simulink model "diapo_model"  (R2014a)
settings: Solver=ode45  StartTime=0.0  StopTime=0.03  RelTol=1e-3
values from neighbouring files (symbols this model uses):
  C = 4.6e-5    (= 4.6e-05)    [tipe_vars.m]
  K = (pi*Rproj^4*gam*(mu*n)^2)/(8*m*Rbob^2)    (= 2.96114824556e-08)    [tipe_vars.m]
  L0 = 0.0015    [tipe_vars.m]
  Lbob = 0.06    [tipe_vars.m]
  Lproj = 0.025    [tipe_vars.m]
  R = 15    [tipe_vars.m]
  Rbob = 0.015    [tipe_vars.m]
  U0 = 800    [tipe_vars.m]
settings Model: Creator=jackhalford  LastModifiedBy=jackhalford
settings SolverCC: ShapePreserveControl=EnableAll  ZeroCrossControl=DisableAll

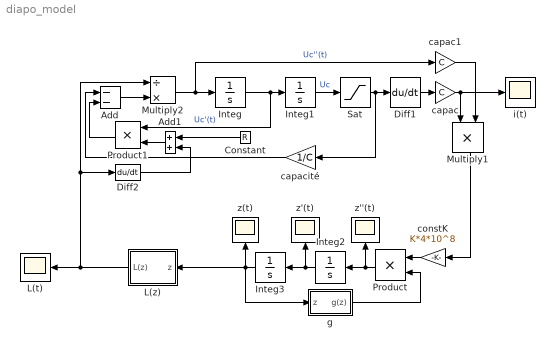
== system diapo_model ==
  Add : Sum  Inputs=--
  Add1 : Sum
  Constant : Constant  Value=R
  Diff1 : Derivative
  Diff2 : Derivative
  Integ : Integrator
  "Integ1 " : Integrator  InitialCondition=-U0
  Integ2 : Integrator  InitialCondition=8
  Integ3 : Integrator  InitialCondition=-(Lbob+Lproj)/2
  L(t) : Scope
      settings: TimeRange=0.003  YMin=-0.0425  YMax=-0.04235
  L(z) : Subsystem
  Multiply1 : Product  Inputs=**
  Multiply2 : Product  Inputs=/*
  Product : Product
  Product1 : Product
  Sat : Saturate  UpperLimit=10000  LowerLimit=-10000
  capac : Gain  Gain=C
  capac1 : Gain  Gain=C
  capacité : Gain  Gain=1/C
  constK : Gain  Gain=K*4*10^8
  g : Subsystem
  i(t) : Scope
      settings: TimeRange=0.005  YMin=0  YMax=80  SaveName=ScopeData17
  z''(t) : Scope
      settings: YMin=1.03225e-09  YMax=1.03675e-09  SaveName=ScopeData3
  z'(t) : Scope
      settings: TimeRange=0.03  YMin=720000  YMax=738000  SaveName=ScopeData13
  z(t) : Scope
      settings: TimeRange=0.003  YMin=-0.0425  YMax=-0.04235  SaveName=ScopeData4
  wires:
  capac/1 -> i(t)/1, Multiply1/1
  Multiply2/1 -> capac1/1, Integ/1  "Uc''(t)"
  Integ/1 -> Product1/1, "Integ1 "/1  "Uc'(t)"
  Product1/1 -> Add/2
  Add/1 -> Multiply2/2
  capacité/1 -> Add/1
  Diff1/1 -> capac/1
  "Integ1 "/1 -> Sat/1  "Uc"
  Sat/1 -> Diff1/1, capacité/1
  Product/1 -> Integ2/1, z''(t)/1
  Integ2/1 -> Integ3/1, z'(t)/1
  Integ3/1 -> z(t)/1, L(z)/1("z "), g/1("z ")
  capac1/1 -> Multiply1/2
  Multiply1/1 -> constK/1
  constK/1 -> Product/1
  g/1(g(z)) -> Product/2
  L(z)/1(L(z)) -> Multiply2/1, Diff2/1, L(t)/1
  Add1/1 -> Product1/2
  Constant/1 -> Add1/1
  Diff2/1 -> Add1/2

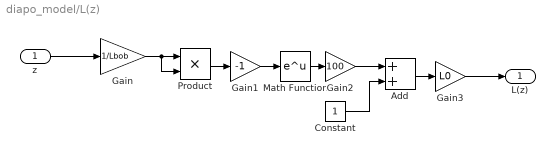
== system diapo_model/L(z) ==
  "z " : Inport
  Add : Sum
  Constant : Constant
  Gain : Gain  Gain=1/Lbob
  Gain1 : Gain  Gain=-1
  Gain2 : Gain  Gain=100
  Gain3 : Gain  Gain=L0
  Math Function : Math  SaturateOnIntegerOverflow=on
  Product : Product
  L(z) : Outport
  wires:
  "z "/1 -> Gain/1
  Gain/1 -> Product/2, Product/1
  Product/1 -> Gain1/1
  Gain1/1 -> Math Function/1
  Math Function/1 -> Gain2/1
  Gain2/1 -> Add/1
  Constant/1 -> Add/2
  Add/1 -> Gain3/1
  Gain3/1 -> L(z)/1

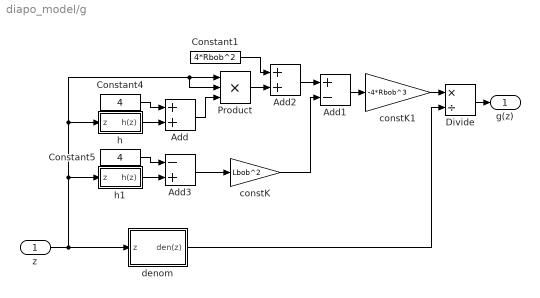
== system diapo_model/g ==
  "z " : Inport
  Add : Sum
  Add1 : Sum  Inputs=+-
  Add2 : Sum
  Add3 : Sum  Inputs=-+
  Constant1 : Constant  Value=4*Rbob^2
  Constant4 : Constant  Value=4
  Constant5 : Constant  Value=4
  Divide : Product  Inputs=*/
  Product : Product  Inputs=3
  constK : Gain  Gain=Lbob^2
  constK1 : Gain  Gain=-4*Rbob^3
  denom : Subsystem
  "h " : Subsystem
  "h1 " : Subsystem
  g(z) : Outport
  wires:
  Add/1 -> Product/3
  "h "/1(h(z)) -> Add/2
  Add2/1 -> Add1/1
  Divide/1 -> g(z)/1
  "z "/1 -> denom/1("z "), "h "/1("z "), Product/2, Product/1, "h1 "/1("z ")
  Constant4/1 -> Add/1
  Product/1 -> Add2/2
  Constant1/1 -> Add2/1
  constK/1 -> Add1/2
  denom/1(den(z)) -> Divide/2
  Constant5/1 -> Add3/1
  "h1 "/1(h(z)) -> Add3/2
  Add3/1 -> constK/1
  constK1/1 -> Divide/1
  Add1/1 -> constK1/1

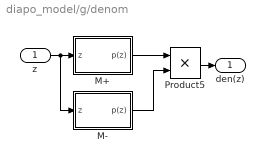
== system diapo_model/g/denom ==
  "z " : Inport
  M+ : Subsystem
  M- : Subsystem
  Product5 : Product
  den(z) : Outport
  wires:
  "z "/1 -> M-/1("z "), M+/1("z ")
  M+/1(p(z)) -> Product5/1
  M-/1(p(z)) -> Product5/2
  Product5/1 -> den(z)/1

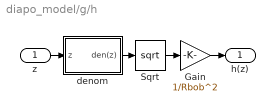
== system diapo_model/g/h  ==
  "z " : Inport
  Gain : Gain  Gain=1/Rbob^2
  Sqrt : Sqrt  SaturateOnIntegerOverflow=on
  denom : Subsystem
  h(z) : Outport
  wires:
  "z "/1 -> denom/1("z ")
  denom/1(den(z)) -> Sqrt/1
  Sqrt/1 -> Gain/1
  Gain/1 -> h(z)/1

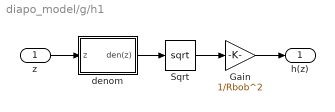
== system diapo_model/g/h1  ==
  "z " : Inport
  Gain : Gain  Gain=1/Rbob^2
  Sqrt : Sqrt  SaturateOnIntegerOverflow=on
  denom : Subsystem
  h(z) : Outport
  wires:
  "z "/1 -> denom/1("z ")
  denom/1(den(z)) -> Sqrt/1
  Sqrt/1 -> Gain/1
  Gain/1 -> h(z)/1

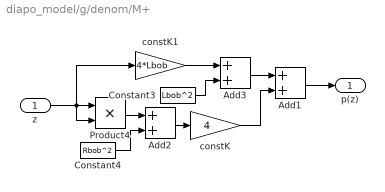
== system diapo_model/g/denom/M+ ==
  "z " : Inport
  Add1 : Sum
  Add2 : Sum
  Add3 : Sum
  Constant3 : Constant  Value=Lbob^2
  Constant4 : Constant  Value=Rbob^2
  Product4 : Product
  constK : Gain  Gain=4
  constK1 : Gain  Gain=4*Lbob
  p(z) : Outport
  wires:
  Product4/1 -> Add2/1
  Constant4/1 -> Add2/2
  Add2/1 -> constK/1
  constK1/1 -> Add3/1
  Constant3/1 -> Add3/2
  "z "/1 -> constK1/1, Product4/2, Product4/1
  Add3/1 -> Add1/1
  constK/1 -> Add1/2
  Add1/1 -> p(z)/1

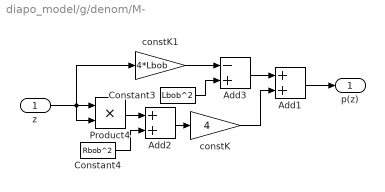
== system diapo_model/g/denom/M- ==
  "z " : Inport
  Add1 : Sum
  Add2 : Sum
  Add3 : Sum  Inputs=-+
  Constant3 : Constant  Value=Lbob^2
  Constant4 : Constant  Value=Rbob^2
  Product4 : Product
  constK : Gain  Gain=4
  constK1 : Gain  Gain=4*Lbob
  p(z) : Outport
  wires:
  Product4/1 -> Add2/1
  Constant4/1 -> Add2/2
  Add2/1 -> constK/1
  constK1/1 -> Add3/1
  Constant3/1 -> Add3/2
  "z "/1 -> constK1/1, Product4/2, Product4/1
  Add3/1 -> Add1/1
  constK/1 -> Add1/2
  Add1/1 -> p(z)/1

== system diapo_model/g/h /denom ==
  "z " : Inport
  M+ : Subsystem
  M- : Subsystem
  Product5 : Product
  den(z) : Outport
  wires:
  "z "/1 -> M-/1("z "), M+/1("z ")
  M+/1(p(z)) -> Product5/1
  M-/1(p(z)) -> Product5/2
  Product5/1 -> den(z)/1

== system diapo_model/g/h1 /denom ==
  "z " : Inport
  M+ : Subsystem
  M- : Subsystem
  Product5 : Product
  den(z) : Outport
  wires:
  "z "/1 -> M-/1("z "), M+/1("z ")
  M+/1(p(z)) -> Product5/1
  M-/1(p(z)) -> Product5/2
  Product5/1 -> den(z)/1

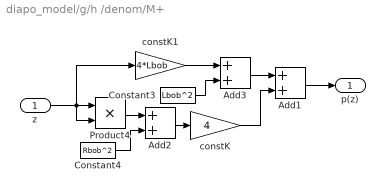
== system diapo_model/g/h /denom/M+ ==
  "z " : Inport
  Add1 : Sum
  Add2 : Sum
  Add3 : Sum
  Constant3 : Constant  Value=Lbob^2
  Constant4 : Constant  Value=Rbob^2
  Product4 : Product
  constK : Gain  Gain=4
  constK1 : Gain  Gain=4*Lbob
  p(z) : Outport
  wires:
  Product4/1 -> Add2/1
  Constant4/1 -> Add2/2
  Add2/1 -> constK/1
  constK1/1 -> Add3/1
  Constant3/1 -> Add3/2
  "z "/1 -> constK1/1, Product4/2, Product4/1
  Add3/1 -> Add1/1
  constK/1 -> Add1/2
  Add1/1 -> p(z)/1

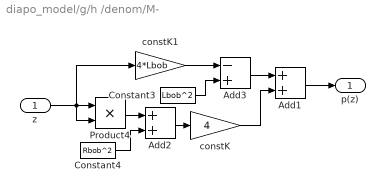
== system diapo_model/g/h /denom/M- ==
  "z " : Inport
  Add1 : Sum
  Add2 : Sum
  Add3 : Sum  Inputs=-+
  Constant3 : Constant  Value=Lbob^2
  Constant4 : Constant  Value=Rbob^2
  Product4 : Product
  constK : Gain  Gain=4
  constK1 : Gain  Gain=4*Lbob
  p(z) : Outport
  wires:
  Product4/1 -> Add2/1
  Constant4/1 -> Add2/2
  Add2/1 -> constK/1
  constK1/1 -> Add3/1
  Constant3/1 -> Add3/2
  "z "/1 -> constK1/1, Product4/2, Product4/1
  Add3/1 -> Add1/1
  constK/1 -> Add1/2
  Add1/1 -> p(z)/1

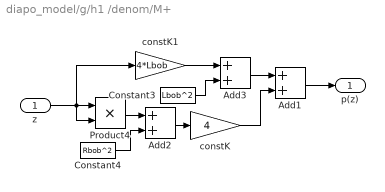
== system diapo_model/g/h1 /denom/M+ ==
  "z " : Inport
  Add1 : Sum
  Add2 : Sum
  Add3 : Sum
  Constant3 : Constant  Value=Lbob^2
  Constant4 : Constant  Value=Rbob^2
  Product4 : Product
  constK : Gain  Gain=4
  constK1 : Gain  Gain=4*Lbob
  p(z) : Outport
  wires:
  Product4/1 -> Add2/1
  Constant4/1 -> Add2/2
  Add2/1 -> constK/1
  constK1/1 -> Add3/1
  Constant3/1 -> Add3/2
  "z "/1 -> constK1/1, Product4/2, Product4/1
  Add3/1 -> Add1/1
  constK/1 -> Add1/2
  Add1/1 -> p(z)/1

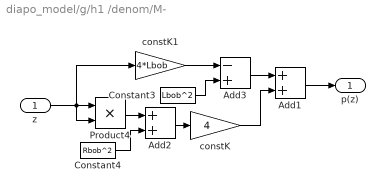
== system diapo_model/g/h1 /denom/M- ==
  "z " : Inport
  Add1 : Sum
  Add2 : Sum
  Add3 : Sum  Inputs=-+
  Constant3 : Constant  Value=Lbob^2
  Constant4 : Constant  Value=Rbob^2
  Product4 : Product
  constK : Gain  Gain=4
  constK1 : Gain  Gain=4*Lbob
  p(z) : Outport
  wires:
  Product4/1 -> Add2/1
  Constant4/1 -> Add2/2
  Add2/1 -> constK/1
  constK1/1 -> Add3/1
  Constant3/1 -> Add3/2
  "z "/1 -> constK1/1, Product4/2, Product4/1
  Add3/1 -> Add1/1
  constK/1 -> Add1/2
  Add1/1 -> p(z)/1
